simulink model "load_from_files"  (R2021b)
settings: Solver=ode4  StartTime=0.0  StopTime=inf  FixedStep=0.001  RelTol=1e-3  EnableMultiTasking=on
model workspace (MATLAB code in the model file):
  | % Add the class folders into the path.
  | addpath src\model
  | addpath src\utils
  | 
  | %% Loading data from files.
  | % Data for supervisor 1.
  | utils = StateMachineUtils;
  | 
  | % From TCT: Load all events' number.
  | utils = utils.loadEventsInAds('resources/tct/ALLEVENT.ADS');
  | 
  | % From TCT: Disabled events in each state.
  | utils = utils.loadDisabledEventsInPdt('resources/tct/supervisor1/DATA_SIMSUP1_MG1.PDT');
  | 
  | % From TCT: Transition matrix.
  | utils = utils.loadTransitionsInAds('resources/tct/supervisor1/SIMSUP1_MG1.ADS');
  | 
  | % Parameters for the block.
  | encodedStates = StateEncoder.encode(utils.statesArray);
  | 
  | transitions = utils.transitions;
  | 
  | allEvents = utils.eventsArray;
libraries: rtlab x2
Description:
  | Model of a simple control system for use iin training.
settings Model: Creator=Paul Baracos  LastModifiedBy=andrerangel
settings SolverCC: AlgebraicLoopSolver=TrustRegion
settings DataIOCC: LimitDataPoints=on  SaveFormat=Array  SignalLoggingSaveFormat=ModelDataLogs  SaveOutput=off  SaveTime=off  ReturnWorkspaceOutputs=off  SignalLoggingName=sigsOut
settings OptimizationCC: BlockReduction=off  BooleanDataType=off  OptimizeBlockIOStorage=off  BufferReuse=off  ExpressionFolding=off  LocalBlockOutputs=off  InitFltsAndDblsToZero=on  LifeSpan=inf
settings DebuggingCC: SaveWithParameterizedLinksMsg=none  UnderspecifiedInitializationDetection=Classic  MergeDetectMultiDrivingBlocksExec=none  SignalResolutionControl=TryResolveAllWithWarning  MultiTaskDSMMsg=warning  MultiTaskCondExecSysMsg=none  FcnCallInpInsideContextMsg=warning  SFUnexpectedBacktrackingDiag=warning  SFNoUnconditionalDefaultTransitionDiag=warning  SFExecutionAtInitializationDiag=none  SFMachineParentedDataDiag=warning  ArithmeticOperatorsInVariantConditions=warning
settings HardwareCC: ProdBitPerPointer=32  ProdBitPerSizeT=32  ProdBitPerPtrDiffT=32  ProdLargestAtomicFloat=None  ProdIntDivRoundTo=Undefined  ProdEndianess=Unspecified  ProdWordSize=32  ProdHWDeviceType=32-bit Generic  TargetUnknown=on
settings ModelReferenceCC: PropagateSignalLabelsOutOfModel=off
settings SFSimCC: SimUseLocalCustomCode=off  CustomCodeUndefinedFunction=UseInterfaceOnly
settings RTWCC: RTWUseLocalCustomCode=off
settings CodeAppCC: StateflowObjectComments=on
settings GRTTargetCC: TargetFcnLib=ansi_tfl_tmw.mat  TargetLangStandard=C89/C90 (ANSI)  CombineOutputUpdateFcns=off  GRTInterface=on
settings ConfigComp: CovMetricSettings=dw  CovSaveCumulativeToWorkspaceVar=on  CovSaveSingleToWorkspaceVar=on  CovExternalEMLEnable=off

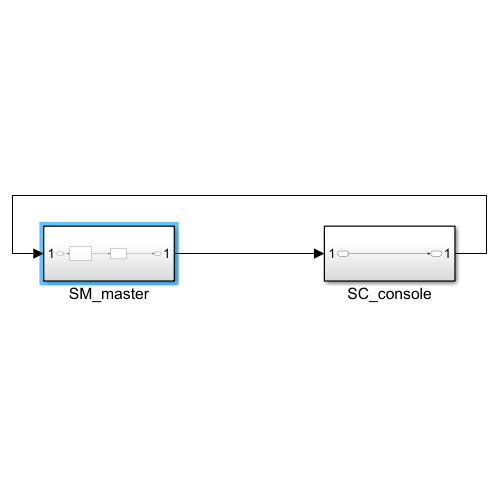
[thumbnail: Simulink's stored preview of the top-level diagram]
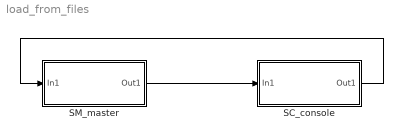
== system load_from_files ==
  SC_console : Subsystem
  SM_master : Subsystem
  wires:
  SM_master/1(Out1) -> SC_console/1(In1)
  SC_console/1(Out1) -> SM_master/1(In1)

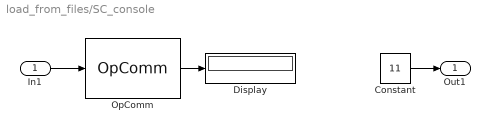
== system load_from_files/SC_console ==
  In1 : Inport
  Constant : Constant  Value=11
  Display : Display
  OpComm : rtlab/OpComm  nbport=1  groupe_acq=1  subsys_rate=0  st=0  Synchronization=on  Interpolation=on  Threshold=1.0  Missed_Data=off  Sim_Time=off  Samples=off  dynSigOut=off  from_console=0  warning_done=off  writeOpCommFile=off  Offset=off
      settings: SourceProductName=RT-LAB
  Out1 : Outport
  wires:
  In1/1 -> OpComm/1
  OpComm/1 -> Display/1
  Constant/1 -> Out1/1

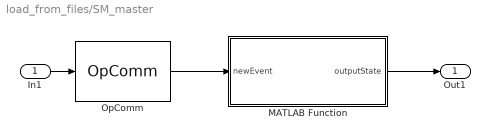
== system load_from_files/SM_master ==
  In1 : Inport
  MATLAB Function : MATLAB Function  TreatAsAtomicUnit=on
  OpComm : rtlab/OpComm  nbport=1  groupe_acq=1  subsys_rate=0  st=0  Synchronization=on  Interpolation=on  Threshold=1.0  Missed_Data=off  Sim_Time=off  Samples=off  dynSigOut=off  from_console=1  warning_done=off  writeOpCommFile=off  Offset=off
      settings: SourceProductName=RT-LAB
  Out1 : Outport
  wires:
  In1/1 -> OpComm/1
  OpComm/1 -> MATLAB Function/1(newEvent)
  MATLAB Function/1(outputState) -> Out1/1

== matlab function load_from_files/SM_master/MATLAB Function ==
  data: newEvent input; outputState output; allEvents parameter; transitions parameter; encodedStates parameter
function outputState  = stateMachine(newEvent, allEvents, transitions, encodedStates)
% State Machine with parameters from files.

% Initialize a persistent object. Its value will not be erased as this
% block finishes.
persistent stateMachine

% Assign the persistent object to the StateMachine class with data passed
% as parameters.
if (isempty(stateMachine))
    statesArray = StateEncoder.decode(encodedStates);                        
    stateMachine = StateMachine(statesArray, transitions, allEvents);
end

stateMachine.inputEvent = newEvent;
outputState = double(stateMachine.currentState.number);
% isActiveArray = stateMachine.currentState.activeEvents;
% eventsNumber = stateMachine.eventsArray;
